simulink model "LQT_konvensional_simulink"  (R2017a)
settings: Solver=VariableStepAuto  StartTime=0.0  StopTime=10.0  RelTol=1e-3
values from neighbouring files (symbols this model uses):
  A = [0 1 0 0 0 ... (first row only)    [DLQR_refluks_konsen.m]    (also in LQT_konvensional_DARE.m = [0 1 0; NARX_MLP.m = eye(na,na))
  B = [0;0;0;0;1]    [DLQR_refluks_konsen.m]    (also in LQT_konvensional_DARE.m = [0;0;1]; NARX_MLP.m = zeros(na,1))
  C = [-b5*a0 -b4*a0 a3-b3*a0 a2-b2*a0 a1-b1*a0]    [DLQR_refluks_konsen.m]    (also in LQT_konvensional_DARE.m = [-b3*a0 a2-b2*a0 a1-b1*a0]; NARX_MLP.m = zeros(1,na))
  Kv = inv(sqrt(discount_fac)*B'*P*sqrt(discount_fac)*B+R)*sqrt(discount_fac)*B'    [DLQR_refluks_konsen.m]    (also in LQT_konvensional_DARE.m = inv(B'*P_dare*B+R)*B')
  Q = 1.025    [DLQR_refluks_konsen.m]    (also in LQT_konvensional_DARE.m = eye(3))
  Q1 = [C'*Q*C -C'*Q;-Q*C Q]    [DLQR_refluks_konsen.m]
undefined symbols (not defined in the file or in its folder): K1_dare, K1v, K2_dare, K2v, K3_dare, K3v, K4_dare, K4v, K5_dare, K5v, K_dare, Q2, Q3, Q4, Q5
settings Model: Creator=HP  LastModifiedBy=HP

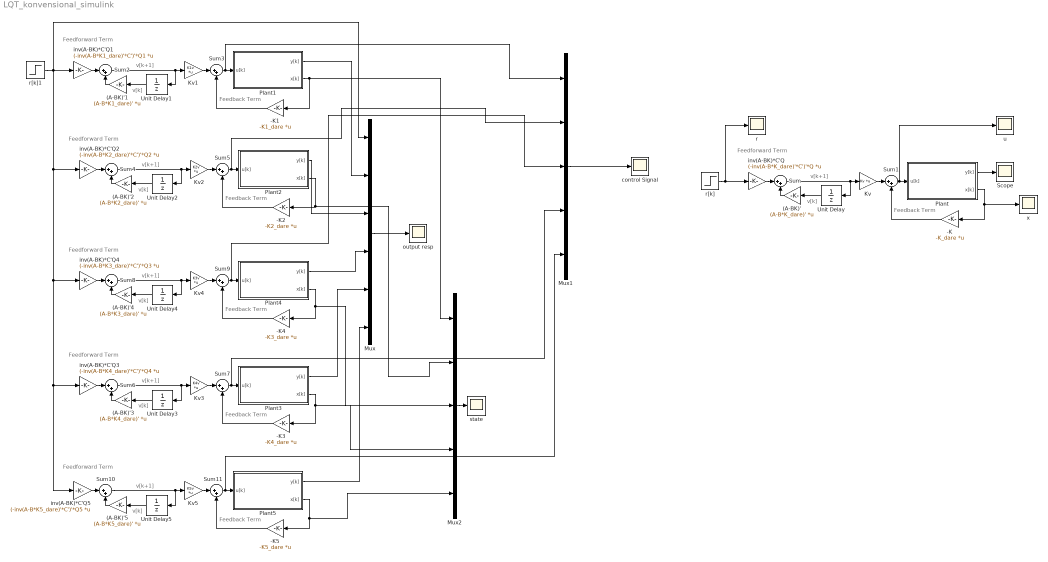
== system LQT_konvensional_simulink ==
  note: v[k+1]
  note: Feedback Term
  note: Feedforward Term
  note: v[k]
  note: v[k+1]
  note: Feedback Term
  note: Feedforward Term
  note: v[k]
  note: v[k+1]
  note: Feedback Term
  note: Feedforward Term
  note: v[k]
  note: v[k+1]
  note: Feedback Term
  note: Feedforward Term
  note: v[k]
  note: v[k+1]
  note: Feedback Term
  note: Feedforward Term
  note: v[k]
  note: v[k+1]
  note: Feedback Term
  note: Feedforward Term
  note: v[k]
  (A-BK)' : Gain  Gain=(A-B*K_dare)'  Multiplication=Matrix(K*u)
  (A-BK)'1 : Gain  Gain=(A-B*K1_dare)'  Multiplication=Matrix(K*u)
  (A-BK)'2 : Gain  Gain=(A-B*K2_dare)'  Multiplication=Matrix(K*u)
  (A-BK)'3 : Gain  Gain=(A-B*K4_dare)'  Multiplication=Matrix(K*u)
  (A-BK)'4 : Gain  Gain=(A-B*K3_dare)'  Multiplication=Matrix(K*u)
  (A-BK)'5 : Gain  Gain=(A-B*K5_dare)'  Multiplication=Matrix(K*u)
  -K : Gain  Gain=-K_dare  Multiplication=Matrix(K*u)
  -K1 : Gain  Gain=-K1_dare  Multiplication=Matrix(K*u)
  -K2 : Gain  Gain=-K2_dare  Multiplication=Matrix(K*u)
  -K3 : Gain  Gain=-K4_dare  Multiplication=Matrix(K*u)
  -K4 : Gain  Gain=-K3_dare  Multiplication=Matrix(K*u)
  -K5 : Gain  Gain=-K5_dare  Multiplication=Matrix(K*u)
  Kv : Gain  Gain=Kv  Multiplication=Matrix(K*u)
  Kv1 : Gain  Gain=K1v  Multiplication=Matrix(K*u)
  Kv2 : Gain  Gain=K2v  Multiplication=Matrix(K*u)
  Kv3 : Gain  Gain=K4v  Multiplication=Matrix(K*u)
  Kv4 : Gain  Gain=K3v  Multiplication=Matrix(K*u)
  Kv5 : Gain  Gain=K5v  Multiplication=Matrix(K*u)
  Mux : Mux  Inputs=6
  Mux1 : Mux  Inputs=5
  Mux2 : Mux  Inputs=5
  Plant : Subsystem
  Plant1 : Subsystem
  Plant2 : Subsystem
  Plant3 : Subsystem
  Plant4 : Subsystem
  Plant5 : Subsystem
  Scope : Scope
  Sum{,1..11} (12 alike) : Sum  Inputs=|++
  Unit Delay{,1..5} (6 alike) : UnitDelay  SampleTime=-1
  control Signal : Scope
  inv(A-BK)*C'Q : Gain  Gain=(-inv(A-B*K_dare)'*C')'*Q  Multiplication=Matrix(K*u)
  inv(A-BK)*C'Q1 : Gain  Gain=(-inv(A-B*K1_dare)'*C')'*Q1  Multiplication=Matrix(K*u)
  inv(A-BK)*C'Q2 : Gain  Gain=(-inv(A-B*K2_dare)'*C')'*Q2  Multiplication=Matrix(K*u)
  inv(A-BK)*C'Q3 : Gain  Gain=(-inv(A-B*K4_dare)'*C')'*Q4  Multiplication=Matrix(K*u)
  inv(A-BK)*C'Q4 : Gain  Gain=(-inv(A-B*K3_dare)'*C')'*Q3  Multiplication=Matrix(K*u)
  inv(A-BK)*C'Q5 : Gain  Gain=(-inv(A-B*K5_dare)'*C')'*Q5  Multiplication=Matrix(K*u)
  output resp : Scope
  r : Scope
  r[k] : Step  Time=[0;0;0]  After=[1;1;1]  SampleTime=0
  r[k]1 : Step  Time=[0;0;0]  After=[1;1;1]  SampleTime=0
  state : Scope
  u : Scope
  x : Scope
  wires:
  Plant/2(x[k]) -> x/1, -K/1
  Sum1/1 -> u/1, Plant/1(u[k])
  -K/1 -> Sum1/2
  Kv/1 -> Sum1/1
  Unit Delay/1 -> (A-BK)'/1
  r[k]/1 -> r/1, inv(A-BK)*C'Q/1
  Sum/1 -> Kv/1, Unit Delay/1
  (A-BK)'/1 -> Sum/2
  inv(A-BK)*C'Q/1 -> Sum/1
  Plant/1(y[k]) -> Scope/1
  inv(A-BK)*C'Q1/1 -> Sum2/1
  (A-BK)'1/1 -> Sum2/2
  Sum2/1 -> Unit Delay1/1, Kv1/1
  Unit Delay1/1 -> (A-BK)'1/1
  Kv1/1 -> Sum3/1
  -K1/1 -> Sum3/2
  Sum3/1 -> Mux1/1, Plant1/1(u[k])
  Plant1/2(x[k]) -> -K1/1, Mux2/1
  Plant2/2(x[k]) -> Mux2/2, -K2/1
  Sum5/1 -> Mux1/2, Plant2/1(u[k])
  -K2/1 -> Sum5/2
  Kv2/1 -> Sum5/1
  Unit Delay2/1 -> (A-BK)'2/1
  Sum4/1 -> Kv2/1, Unit Delay2/1
  (A-BK)'2/1 -> Sum4/2
  inv(A-BK)*C'Q2/1 -> Sum4/1
  inv(A-BK)*C'Q3/1 -> Sum6/1
  (A-BK)'3/1 -> Sum6/2
  Sum6/1 -> Unit Delay3/1, Kv3/1
  Unit Delay3/1 -> (A-BK)'3/1
  Kv3/1 -> Sum7/1
  -K3/1 -> Sum7/2
  Sum7/1 -> Mux1/4, Plant3/1(u[k])
  Plant3/2(x[k]) -> Mux2/4, -K3/1
  Plant4/2(x[k]) -> Mux2/3, -K4/1
  Sum9/1 -> Mux1/3, Plant4/1(u[k])
  -K4/1 -> Sum9/2
  Kv4/1 -> Sum9/1
  Unit Delay4/1 -> (A-BK)'4/1
  Sum8/1 -> Kv4/1, Unit Delay4/1
  (A-BK)'4/1 -> Sum8/2
  inv(A-BK)*C'Q4/1 -> Sum8/1
  Plant5/2(x[k]) -> Mux2/5, -K5/1
  Sum11/1 -> Mux1/5, Plant5/1(u[k])
  -K5/1 -> Sum11/2
  Kv5/1 -> Sum11/1
  Unit Delay5/1 -> (A-BK)'5/1
  r[k]1/1 -> inv(A-BK)*C'Q5/1, inv(A-BK)*C'Q3/1, inv(A-BK)*C'Q4/1, inv(A-BK)*C'Q2/1, Mux/1, inv(A-BK)*C'Q1/1
  Sum10/1 -> Kv5/1, Unit Delay5/1
  (A-BK)'5/1 -> Sum10/2
  inv(A-BK)*C'Q5/1 -> Sum10/1
  Mux/1 -> output resp/1
  Plant1/1(y[k]) -> Mux/2
  Plant2/1(y[k]) -> Mux/3
  Plant4/1(y[k]) -> Mux/4
  Plant3/1(y[k]) -> Mux/5
  Plant5/1(y[k]) -> Mux/6
  Mux2/1 -> state/1
  Mux1/1 -> control Signal/1

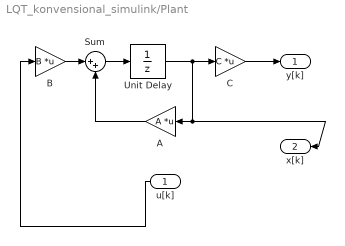
== system LQT_konvensional_simulink/Plant ==
  u[k] : Inport
  A : Gain  Gain=A  Multiplication=Matrix(K*u)
  B : Gain  Gain=B  Multiplication=Matrix(K*u)
  C : Gain  Gain=C  Multiplication=Matrix(K*u)
  Sum : Sum  Inputs=|++
  Unit Delay : UnitDelay  SampleTime=-1
  y[k] : Outport
  x[k] : Outport  Port=2
  wires:
  Sum/1 -> Unit Delay/1
  B/1 -> Sum/1
  Unit Delay/1 -> C/1, x[k]/1, A/1
  u[k]/1 -> B/1
  A/1 -> Sum/2
  C/1 -> y[k]/1

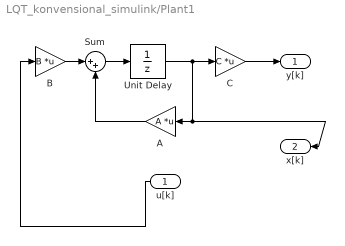
== system LQT_konvensional_simulink/Plant1 ==
  u[k] : Inport
  A : Gain  Gain=A  Multiplication=Matrix(K*u)
  B : Gain  Gain=B  Multiplication=Matrix(K*u)
  C : Gain  Gain=C  Multiplication=Matrix(K*u)
  Sum : Sum  Inputs=|++
  Unit Delay : UnitDelay  SampleTime=-1
  y[k] : Outport
  x[k] : Outport  Port=2
  wires:
  C/1 -> y[k]/1
  A/1 -> Sum/2
  u[k]/1 -> B/1
  Unit Delay/1 -> A/1, x[k]/1, C/1
  B/1 -> Sum/1
  Sum/1 -> Unit Delay/1

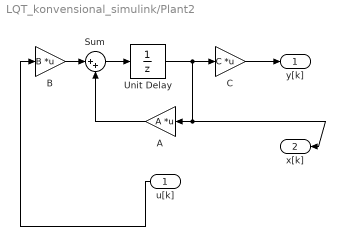
== system LQT_konvensional_simulink/Plant2 ==
  u[k] : Inport
  A : Gain  Gain=A  Multiplication=Matrix(K*u)
  B : Gain  Gain=B  Multiplication=Matrix(K*u)
  C : Gain  Gain=C  Multiplication=Matrix(K*u)
  Sum : Sum  Inputs=|++
  Unit Delay : UnitDelay  SampleTime=-1
  y[k] : Outport
  x[k] : Outport  Port=2
  wires:
  Sum/1 -> Unit Delay/1
  B/1 -> Sum/1
  Unit Delay/1 -> C/1, x[k]/1, A/1
  u[k]/1 -> B/1
  A/1 -> Sum/2
  C/1 -> y[k]/1

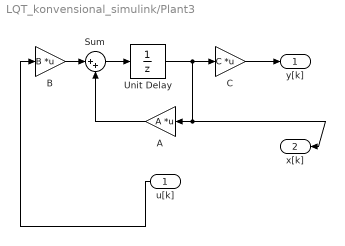
== system LQT_konvensional_simulink/Plant3 ==
  u[k] : Inport
  A : Gain  Gain=A  Multiplication=Matrix(K*u)
  B : Gain  Gain=B  Multiplication=Matrix(K*u)
  C : Gain  Gain=C  Multiplication=Matrix(K*u)
  Sum : Sum  Inputs=|++
  Unit Delay : UnitDelay  SampleTime=-1
  y[k] : Outport
  x[k] : Outport  Port=2
  wires:
  C/1 -> y[k]/1
  A/1 -> Sum/2
  u[k]/1 -> B/1
  Unit Delay/1 -> A/1, x[k]/1, C/1
  B/1 -> Sum/1
  Sum/1 -> Unit Delay/1

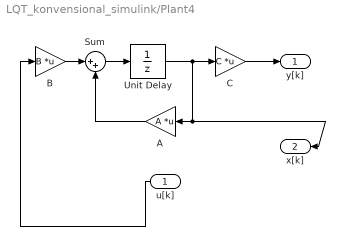
== system LQT_konvensional_simulink/Plant4 ==
  u[k] : Inport
  A : Gain  Gain=A  Multiplication=Matrix(K*u)
  B : Gain  Gain=B  Multiplication=Matrix(K*u)
  C : Gain  Gain=C  Multiplication=Matrix(K*u)
  Sum : Sum  Inputs=|++
  Unit Delay : UnitDelay  SampleTime=-1
  y[k] : Outport
  x[k] : Outport  Port=2
  wires:
  Sum/1 -> Unit Delay/1
  B/1 -> Sum/1
  Unit Delay/1 -> C/1, x[k]/1, A/1
  u[k]/1 -> B/1
  A/1 -> Sum/2
  C/1 -> y[k]/1

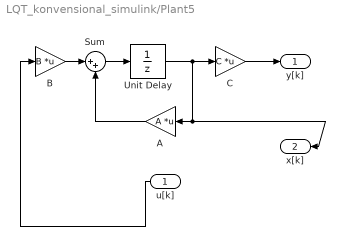
== system LQT_konvensional_simulink/Plant5 ==
  u[k] : Inport
  A : Gain  Gain=A  Multiplication=Matrix(K*u)
  B : Gain  Gain=B  Multiplication=Matrix(K*u)
  C : Gain  Gain=C  Multiplication=Matrix(K*u)
  Sum : Sum  Inputs=|++
  Unit Delay : UnitDelay  SampleTime=-1
  y[k] : Outport
  x[k] : Outport  Port=2
  wires:
  Sum/1 -> Unit Delay/1
  B/1 -> Sum/1
  Unit Delay/1 -> C/1, x[k]/1, A/1
  u[k]/1 -> B/1
  A/1 -> Sum/2
  C/1 -> y[k]/1
